simulink model "UnmodifiedMotoHawkModel"  (R2016a)
settings: Solver=ode4  SolverMode=SingleTasking  StartTime=0.0  StopTime=10.0  FixedStep=0.001  RelTol=1e-3
values from neighbouring files (symbols this model uses):
  engineblendfactormap = [0 0 0 0 0 0 0 0 0 0 0 0 ... (420 elements, 21x20)]    [blendfactorvariables.mat]
  motorblendfactormap = [1 1 1 1 1 1 1 1 1 1 1 1 ... (420 elements, 21x20)]    [blendfactorvariables.mat]
  v = [0 5 10 15 20 25 30 35 40 45 50 55 ... (21 elements, 1x21)]    [blendfactorvariables.mat]
  x = [0 1 2 3 4 5 6 7 8 9 10 11 ... (20 elements, 1x20)]    [blendfactorvariables.mat]
undefined symbols (not defined in the file or in its folder): ECU565, motohawk_build_version, motohawk_trunc_name, motohawk_vardec_path
libraries: MotoHawk_lib x58
(part 2 of 2)

== stateflow chart UnmodifiedMotoHawkModel/Function-Call Subsystem/Controller/Engine State Logic/Engine State Logic ==
  state EngineCrankState
    en,du:
    EngineState=2;
    EngineCrankTime=temporalCount(sec);
  state EngineOff
    en:EngineState=1;
  state EngineStartFail
    en:EngineState=5;
  state EngineOn
    en:EngineState=4;
  state EngineWarmup
    en,du:
    EngineState=3;
    EngineWarmUpTime=temporalCount(sec);
  (default) -> EngineOff
  EngineOff -> EngineCrankState : [EngineCrank==1 && EngineKill==0]
  EngineStartFail -> EngineOff
  EngineCrankState -> EngineStartFail [order 2] : [RPM<=800&&EngineCrankTime>1]
  EngineCrankState -> EngineWarmup [order 1] : [RPM>800&&EngineCrankTime>0.6]
  EngineOn -> EngineOff : [RPM<50 || EngineKill==1]
  EngineWarmup -> EngineStartFail [order 2] : [RPM<500 && EngineWarmUpTime>1]
  EngineWarmup -> EngineOn [order 1] : [RPM>=500 && EngineWarmUpTime>1]
  data: RPM input; EngineKill input; EngineCrank input; EngineState output; time local; EngineCrankTime local; EngineWarmUpTime local

== stateflow chart UnmodifiedMotoHawkModel/Function-Call Subsystem/Controller/Throttle//Torque Request/Engine Throttle Request ==
  state ElectricSolo
    du:EngineThrottleReq=0;
  state BlendingMode
    state EngineState23
      en,du:
      EngineThrottleReq=7.5;
    state OtherStates
      en,du:
      EngineThrottleReq=APP*EngineBlendFactor;
    EngineState23 -> (junction 75) : [EngineState~=2||EngineState~=3]
    (junction 75) -> EngineState23 [order 1] : [EngineState==2||EngineState==3]
    (default) -> OtherStates
    (junction 75) -> OtherStates [order 2] : [EngineState~=2||EngineState~=3]
    OtherStates -> (junction 75) : [EngineState==2||EngineState==3]
  state EngineSole
    du:EngineThrottleReq=APP;
  (junction 74) -> ElectricSolo [order 1] : [Driving_Mode==1]
  (junction 74) -> BlendingMode [order 2] : [Driving_Mode==2]
  BlendingMode -> (junction 74) : [Driving_Mode~=2]
  (junction 74) -> EngineSole [order 3] : [Driving_Mode==3]
  EngineSole -> (junction 74) : [Driving_Mode~=3]
  ElectricSolo -> (junction 74) : [Driving_Mode~=1]
  (default) -> ElectricSolo
  data: Driving_Mode input; EngineBlendFactor input; APP input; EngineState input; EngineThrottleReq output

== stateflow chart UnmodifiedMotoHawkModel/Function-Call Subsystem/Controller/Driving Mode/Driving Mode Controller ==
  state DM
    state EngineSolo
      du:Driving_Mode=3;
    state BlendingMode
      du:Driving_Mode=2;
    state ElectricSolo
      du:Driving_Mode=1;
    EngineSolo -> (junction 14) : [Engine_On_Switch==0||Motor_On_Switch==1]
    (junction 14) -> EngineSolo [order 1] : [Engine_On_Switch==1&&Motor_On_Switch==0&&v<1]
    (junction 14) -> ElectricSolo [order 3] : [Engine_On_Switch==0&&Motor_On_Switch==1&&v<1]
    BlendingMode -> (junction 14) : [Engine_On_Switch==1||Motor_On_Switch==1]
    (junction 14) -> BlendingMode [order 2] : [Engine_On_Switch==0&&Motor_On_Switch==0&&v<1]
    ElectricSolo -> (junction 14) : [Engine_On_Switch==1||Motor_On_Switch==0]
    (default) -> ElectricSolo
  state Nothing
  (default) -> Nothing
  Nothing -> DM : [v<=1]
  DM -> Nothing : [v>1]
  data: Engine_On_Switch input; Motor_On_Switch input; v input; Driving_Mode output

== stateflow chart UnmodifiedMotoHawkModel/Function-Call Subsystem/Controller/Throttle//Torque Request/Motor Throttle Request ==
  state EngineSolo
    du:MotorTorqueReq=0;
  state BlendingMode
    du:MotorTorqueReq=APP*MotorBlendFactor;
  state ElectricSolo
    du:MotorTorqueReq=APP;
  (junction 79) -> ElectricSolo [order 1] : [Driving_Mode==1]
  (junction 79) -> EngineSolo [order 3] : [Driving_Mode==3]
  ElectricSolo -> (junction 79) : [Driving_Mode~=1]
  EngineSolo -> (junction 79) : [Driving_Mode~=3]
  BlendingMode -> (junction 79) : [Driving_Mode~=2]
  (junction 79) -> BlendingMode [order 2] : [Driving_Mode==2]
  (default) -> ElectricSolo
  data: Driving_Mode input; APP input; MotorBlendFactor input; MotorTorqueReq output

== stateflow chart UnmodifiedMotoHawkModel/Function-Call Subsystem/Controller/Engine Start//Stop/EnginE Kill ==
  state EngineSolo
    du:EngineKill=0;AutomaticCrank=0;
  state BlendingMode
    state a
      du:EngineKill=0;
      state c
        du:AutomaticCrank=1;
      state c1
        du:AutomaticCrank=0;
      (default) -> c
      c1 -> c : [EngineState==1]
      c -> c1 : [EngineState~=1]
    state b
      du:EngineKill=1;AutomaticCrank=0;
    (junction 13) -> a [order 1] : [EngineBlendFactor>0.01]
    a -> (junction 13) : [EngineBlendFactor<=0.01]
    b -> (junction 13) : [EngineBlendFactor>0.01]
    (junction 13) -> b [order 2] : [EngineBlendFactor<=0.01]
    (default) -> a
  state ElectricSolo
    du:EngineKill=1;AutomaticCrank=0;
  (junction 3) -> EngineSolo [order 3] : [Driving_Mode==3]
  EngineSolo -> (junction 3) : [Driving_Mode~=3]
  (junction 3) -> ElectricSolo [order 1] : [Driving_Mode==1]
  (junction 3) -> BlendingMode [order 2] : [Driving_Mode==2]
  BlendingMode -> (junction 3) : [Driving_Mode~=2]
  ElectricSolo -> (junction 3) : [Driving_Mode~=1]
  (default) -> ElectricSolo
  data: Driving_Mode input; EngineBlendFactor input; EngineKill output; EngineState input; AutomaticCrank output

== stateflow chart UnmodifiedMotoHawkModel/Function-Call Subsystem/Controller/Engine Start//Stop/Manual Crank ==
  state ElectricSolo
    du:ManualCrank=0;
  state EngineSolo
    state On
      du:ManualCrank=1;
    state Off
      du:ManualCrank=0;
    (junction 14) -> On [order 1] : [CrankSwitch==1]
    (junction 14) -> Off [order 2] : [CrankSwitch==0]
    Off -> (junction 14) : [CrankSwitch~=0]
    On -> (junction 14) : [CrankSwitch~=1]
    (default) -> Off
  state BlendingMode
    du:ManualCrank=0;
  (junction 1) -> EngineSolo [order 3] : [Driving_Mode==3]
  (junction 1) -> ElectricSolo [order 1] : [Driving_Mode==1]
  BlendingMode -> (junction 1) : [Driving_Mode~=2]
  EngineSolo -> (junction 1) : [Driving_Mode~=3]
  ElectricSolo -> (junction 1) : [Driving_Mode~=1]
  (junction 1) -> BlendingMode [order 2] : [Driving_Mode==2]
  (default) -> ElectricSolo
  data: Driving_Mode input; CrankSwitch input; ManualCrank output

== stateflow chart UnmodifiedMotoHawkModel/Function-Call Subsystem/Controller/E-motor start//stop model/E-Motor Start//Stop ==
  state BlendingMode
    state B2
      du:Motor_On=0;
      du:Forward_Signal=1;
      du:Reverse_Signal=0;
    state B1
      du:Motor_On=1;
      du:Forward_Signal=1;
      du:Reverse_Signal=0;
    (junction 11) -> B2 [order 2] : [MotorBlendFactor<=0.01]
    (junction 11) -> B1 [order 1] : [MotorBlendFactor>0.01]
    B1 -> (junction 11) : [MotorBlendFactor<=0.01]
    B2 -> (junction 11) : [MotorBlendFactor>0.01]
    (default) -> B2
  state ElectricSolo
    du:Motor_On=1;
    du:Forward_Signal=ForwardSwitch;
    du:Reverse_Signal=ReverseSwitch;
  state EngineSolo
    du:Motor_On=0;
    du:Forward_Signal=0;
    du:Reverse_Signal=0;
  (default) -> ElectricSolo
  (junction 5) -> BlendingMode [order 2] : [Driving_Mode==2]
  (junction 5) -> ElectricSolo [order 1] : [Driving_Mode==1]
  ElectricSolo -> (junction 5) : [Driving_Mode~=1]
  BlendingMode -> (junction 5) : [Driving_Mode~=2]
  (junction 5) -> EngineSolo [order 3] : [Driving_Mode==3]
  EngineSolo -> (junction 5) : [Driving_Mode~=3]
  data: Driving_Mode input; MotorBlendFactor input; ForwardSwitch input; ReverseSwitch input; Motor_On output; Forward_Signal output; Reverse_Signal output

== stateflow chart UnmodifiedMotoHawkModel/Function-Call Subsystem/Controller/Stepper Motor/Chart ==
  state Step3
    en:T3=T;
    du:Q1=1;
    Q2=0;
    Q3=0;
    Q4=1;
  state Step4
    en:T4=T;
    du:Q1=0;
    Q2=0;
    Q3=0;
    Q4=1;
  state Step2
    en:T2=T;
    du:Q1=1;
    Q2=0;
    Q3=0;
    Q4=0;
  state Step1
    en:T1=T;
    du:Q1=1;
    Q2=0;
    Q3=1;
    Q4=0;
  state Step5
    en:T5=T;
    du:Q1=0;
    Q2=1;
    Q3=0;
    Q4=1;
  state Step8
    en:T8=T;
    du:Q1=0;
    Q2=0;
    Q3=1;
    Q4=0;
  state Step7
    en:T7=T;
    du:Q1=0;
    Q2=1;
    Q3=1;
    Q4=0;
  state Step6
    en:T6=T;
    du:Q1=0;
    Q2=1;
    Q3=0;
    Q4=0;
  Step4 -> Step3 [order 2] : [diff<=-1&&(T-T4)>5]
  Step2 -> Step3 [order 1] : [diff>=1&&(T-T2)>5]
  Step3 -> Step4 [order 1] : [diff>=1&&(T-T3)>5]
  Step1 -> Step2 [order 1] : [diff>=1&&(T-T1)>5]
  Step5 -> Step4 [order 2] : [diff<=-1&&(T-T5)>5]
  Step3 -> Step2 [order 2] : [diff<=-1&&(T-T3)>5]
  Step4 -> Step5 [order 1] : [diff>=1&&(T-T4)>5]
  Step2 -> Step1 [order 2] : [diff<=-1&&(T-T2)>5]
  (default) -> Step1
  Step6 -> Step5 [order 2] : [diff<=-1&&(T-T6)>5]
  Step1 -> Step8 [order 2] : [diff<=-1&&(T-T1)>5]
  Step5 -> Step6 [order 1] : [diff>=1&&(T-T5)>5]
  Step8 -> Step1 [order 1] : [diff>=1&&(T-T8)>5]
  Step7 -> Step8 [order 1] : [diff>=1&&(T-T7)>5]
  Step8 -> Step7 [order 2] : [diff<=-1&&(T-T8)>5]
  Step6 -> Step7 [order 1] : [diff>=1&&(T-T6)>5]
  Step7 -> Step6 [order 2] : [diff<=-1&&(T-T7)>5]
  data: diff input; Q1 output; Q2 output; Q3 output; Q4 output; T input; T3 local; T4 local; T2 local; T1 local; T5 local; T8 local; T7 local; T6 local
